simulink model "STFT_Log_IP"  (R2023b)
settings: Solver=VariableStepAuto  StartTime=0.0  StopTime=5*2*2048*15/fs  RelTol=1e-3
values from neighbouring files (symbols this model uses):
  f = 14.5e6    (= 14500000)    [startup.m]
  fs = 16e6    (= 16000000)    [startup.m]
  N = 2048    [startup.m]
libraries: hdlBasic x55, hdlDSPIP x1, hdlsllib x1, dspsrcs4 x1, vmcUtilities x1
settings Model: Creator=andre  LastModifiedBy=andre

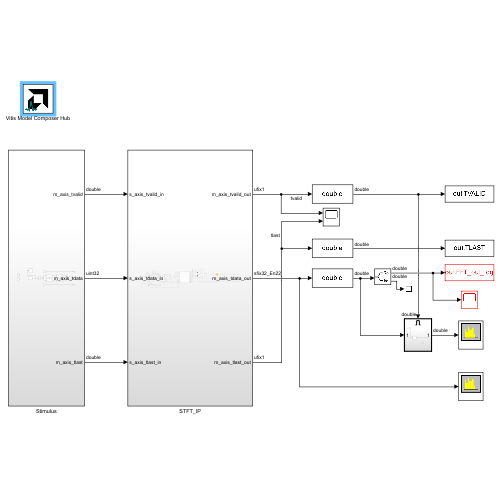
[thumbnail: Simulink's stored preview of the top-level diagram]
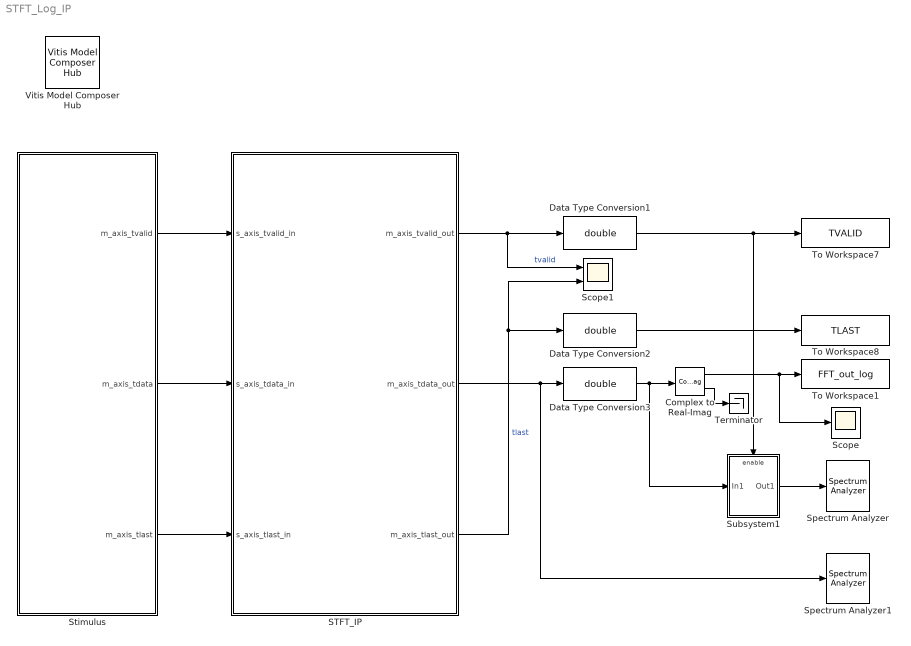
== system STFT_Log_IP ==
  Complex to Real-Imag : ComplexToRealImag
  Data Type Conversion1 : DataTypeConversion  OutDataTypeStr=double  RndMeth=Floor
  Data Type Conversion2 : DataTypeConversion  OutDataTypeStr=double  RndMeth=Floor
  Data Type Conversion3 : DataTypeConversion  OutDataTypeStr=double  RndMeth=Floor
  STFT_IP : Subsystem
  Scope : Scope
  Scope1 : Scope  NumInputPorts=2
  Spectrum Analyzer : SpectrumAnalyzer  WindowPosition=[2193.000000,-144.000000,800.000000,500.000000,]  ScopeFrameLocation=window  InputDomain=Frequency  ViewType=Spectrum and spectrogram  SampleRate=16000000  PlotAsTwoSidedSpectrum=off  AxesScaling=Manual  Span=5000  CenterFrequency=2500  StartFrequency=0  AveragingMethod=Exponential  SpectrumUnits=Auto  YLimits=[-192.92718452,-9.62777478]  ColorLimits=[-192.92718452,-9.62777478]  ExpandToolstrip=on  DefaultConfigurationName=spbscopes.SpectrumAnalyzerBlockCfg  IsFrequencyInputMode=1  FrequencyVectorPort=0  FrequencyVectorFromPort=0  FrequencyInputRBWPort=0  FrequencyInputRBWFromPort=0
  Spectrum Analyzer1 : SpectrumAnalyzer  WindowPosition=[2780.000000,-120.000000,800.000000,500.000000,]  ScopeFrameLocation=window  ViewType=Spectrum and spectrogram  SampleRate=16000000  PlotAsTwoSidedSpectrum=off  AxesScaling=Manual  Span=5000  CenterFrequency=2500  StartFrequency=0  AveragingMethod=Exponential  YLimits=[-4.45804472,88.02345412]  ColorLimits=[-4.45804472,88.02345412]  ExpandToolstrip=on  SelectedToolstripTab=spectrumAnalyzerToolstrip.estimationTab  DefaultConfigurationName=spbscopes.SpectrumAnalyzerBlockCfg  IsFrequencyInputMode=1  FrequencyVectorPort=0  FrequencyVectorFromPort=0  FrequencyInputRBWPort=0  FrequencyInputRBWFromPort=0
  Stimulus : Subsystem
  Subsystem1 : Subsystem
  Terminator : Terminator
  To Workspace1 : ToWorkspace  VariableName=FFT_out_log  SampleTime=-1
      settings: Save2DSignal=2-D array (concatenate along first dimension)
  To Workspace7 : ToWorkspace  VariableName=TVALID  SampleTime=1/fs
      settings: Save2DSignal=2-D array (concatenate along first dimension)
  To Workspace8 : ToWorkspace  VariableName=TLAST  SampleTime=1/fs
      settings: Save2DSignal=2-D array (concatenate along first dimension)
  Vitis Model Composer Hub : vmcUtilities/Vitis Model Composer Hub  Tag=genX  CodeGeneration=off  SubsystemName=STFT_IP  DUTSubsystemName=STFT_IP  CompilationType=HDLCompilation  ExportTypeV2=IP Catalog  TargetDirectory=./netlist\ip\STFT_IP\src  exportDesign=on  analyzeDesign=off  validateDesignOnHw=off  ExportType=HDL  IpVendor=xilinx.com  IpLibrary=hls  IpVersion=1.0  IpHWLanguage=Verilog  AieCompilerOptions={}  AieSimulatorOptions={}  CreateTestbench=off  TestbenchStackSize=10  RunRtlSim=off  RunCSim=off  RunAieSim=off  AieSimTimeout=50000  RunAieSimProfiling=off  LaunchVitisAnalyzer=off  PlotOutput=off  RunX86Sim=off  X86SimTimeout=10  GenHwImage=off  GenLibadfXo=on  GenHwValidationCode=off  PlatformType=Not Specified  HwSystemType=Baremetal  HwValidationTarget=hw  ProjDevice=xczu28dr-ffvg1517-2-e  ProjDevicePart=xczu28dr-ffvg1517-2-e  SamplePeriod=-1  ClockFrequency=200  DataPathParallelism=1  xilinxfamily=zynquplusRFSOC  part=xczu28dr  speed=-2-e  package=ffvg1517  directory=./netlist\ip\STFT_IP\src  testbench=off  incr_netlist=off  synthesis_tool=Vivado  clock_wrapper=Clock Enables  dbl_ovrd=According to Block Masks  dcm_input_clock_period=10  sysclk_period=(1/fs)*(1e6)  simulink_period=1/fs  eval_field=0  IPInfoJsonString="{\"HDLSubsystem\":{\"SubsystemName\":\"STFT_IP\",\"IPName\":\"STFT\",\"IPLibrary\":\"VMC\",\"IPVendor\":\"CoRSoC\",\"IPVersion\":\"1.0\",\"TargetDirectory\":\"./netlist\",\"SubsystemDir\":\"./netlist\\\\ip\\\\STFT_IP\"},\"SubsystemTag\":\"HDLNode\"}"  LogFileName=''  NThreads=4
  wires:
  Stimulus/3(m_axis_tlast) -> STFT_IP/3(s_axis_tlast_in)
  Data Type Conversion1/1 -> To Workspace7/1, Subsystem1/Enable
  Subsystem1/1(Out1) -> Spectrum Analyzer/1
  Complex to Real-Imag/2 -> Terminator/1
  Complex to Real-Imag/1 -> To Workspace1/1, Scope/1
  Data Type Conversion3/1 -> Subsystem1/1(In1), Complex to Real-Imag/1
  STFT_IP/2(m_axis_tdata_out) -> Spectrum Analyzer1/1, Data Type Conversion3/1
  STFT_IP/3(m_axis_tlast_out) -> Scope1/2, Data Type Conversion2/1  "tlast"
  STFT_IP/1(m_axis_tvalid_out) -> Data Type Conversion1/1, Scope1/1  "tvalid"
  Data Type Conversion2/1 -> To Workspace8/1
  Stimulus/1(m_axis_tvalid) -> STFT_IP/1(s_axis_tvalid_in)
  Stimulus/2(m_axis_tdata) -> STFT_IP/2(s_axis_tdata_in)

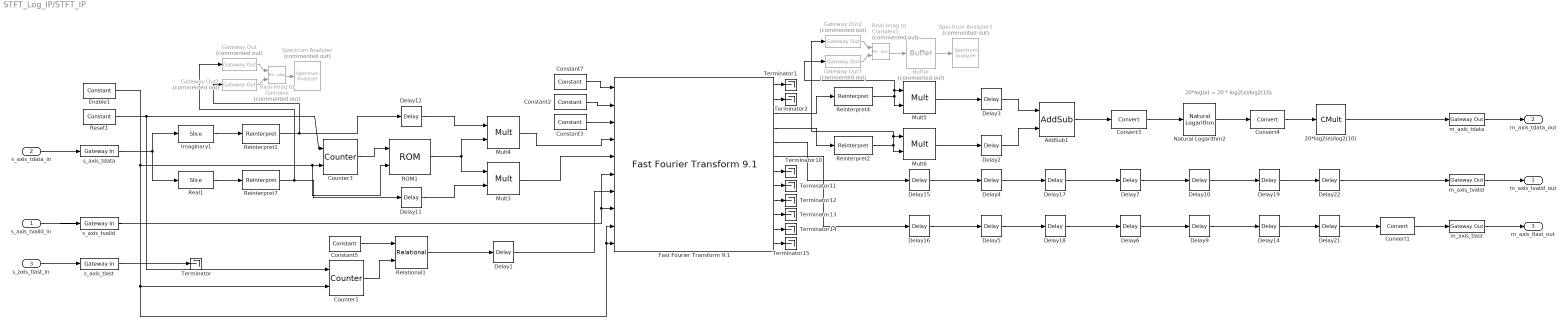
== system STFT_Log_IP/STFT_IP ==
  note: 20*log(x) = 20 * log2(x)/log2(10)
  s_axis_tvalid_in : Inport
  s_axis_tdata_in : Inport  Port=2
  s_axis_tlast_in : Inport  Port=3
  20*log2(e)/log2(10) : hdlBasic/CMult  const=20*1.44269504089/3.32192809489  gui_display_data_type=Fixed-point  const_n_bits=20  const_bin_pt=16  float_type=Single  exp_bits=8  fraction_bits=24  en=off  latency=2  precision=User Defined  arith_type="Signed  (2's comp)"  n_bits=32  bin_pt=32-10  quantization=Truncate  overflow=Saturate  use_behavioral_HDL=off  mem_type=Distributed RAM  pipeline=off  XmcBlockStatus=1  maskContainerNames=tabcontainer1  block_type=cmult  block_config=sysgen:CMult_config
      settings: infoedit=[]
  AddSub1 : hdlBasic/AddSub  mode=Addition  use_carryin=off  use_carryout=off  en=off  latency=1  precision=User Defined  arith_type="Signed  (2's comp)"  n_bits=32  bin_pt=29  quantization=Truncate  overflow=Saturate  use_behavioral_HDL=off  hw_selection=Fabric  pipelined=off  XmcBlockStatus=1  maskContainerNames=tabcontainer1  block_type=addsub  block_config=sysgen:Addsub_config
  Buffer : Buffer  Commented=on  OutputFrames=off
  Constant2 : hdlBasic/Constant  const=0  gui_display_data_type=Fixed-point  arith_type=Unsigned  n_bits=1  bin_pt=0  preci_type=Single  exp_width=8  frac_width=24  explicit_period=on  period=1/fs  XmcBlockStatus=1  maskContainerNames=tabcontainer1  block_type=constant  block_config=sysgen:Constant_config
  Constant3 : hdlBasic/Constant  const=0  gui_display_data_type=Boolean  arith_type=Boolean  n_bits=1  bin_pt=0  preci_type=Single  exp_width=8  frac_width=24  explicit_period=on  period=1/fs  XmcBlockStatus=1  maskContainerNames=tabcontainer1  block_type=constant  block_config=sysgen:Constant_config
  Constant5 : hdlBasic/Constant  const=N-1  gui_display_data_type=Fixed-point  arith_type=Unsigned  n_bits=11  bin_pt=0  preci_type=Single  exp_width=8  frac_width=24  explicit_period=on  period=1/fs  XmcBlockStatus=1  maskContainerNames=tabcontainer1  block_type=constant  block_config=sysgen:Constant_config
  Constant7 : hdlBasic/Constant  const=0  gui_display_data_type=Fixed-point  arith_type=Unsigned  n_bits=12  bin_pt=0  preci_type=Single  exp_width=8  frac_width=24  explicit_period=on  period=1/fs  XmcBlockStatus=1  maskContainerNames=tabcontainer1  block_type=constant  block_config=sysgen:Constant_config
  Convert1 : hdlBasic/Convert  gui_display_data_type=Boolean  arith_type=Boolean  n_bits=16  bin_pt=14  float_type=Single  exp_bits=8  fraction_bits=24  quantization=Truncate  overflow=Wrap  en=off  latency=0  pipeline=off  XmcBlockStatus=1  maskContainerNames=group2  block_type=convert  block_config=sysgen:Convert_config  block_width=595  block_height=885
  Convert3 : hdlBasic/Convert  gui_display_data_type=Floating-point  arith_type=Floating-point  n_bits=16  bin_pt=14  float_type=Single  exp_bits=8  fraction_bits=24  quantization=Truncate  overflow=Wrap  en=off  latency=1  pipeline=off  XmcBlockStatus=1  maskContainerNames=group2  block_type=convert  block_config=sysgen:Convert_config  block_width=595  block_height=885
  Convert4 : hdlBasic/Convert  gui_display_data_type=Fixed-point  arith_type="Signed  (2's comp)"  n_bits=32  bin_pt=32-10  float_type=Single  exp_bits=8  fraction_bits=24  quantization="Round  (unbiased: +/- Inf)"  overflow=Saturate  en=off  latency=1  pipeline=off  XmcBlockStatus=1  maskContainerNames=group2  block_type=convert  block_config=sysgen:Convert_config  block_width=595  block_height=885
  Counter1 : hdlBasic/Counter  cnt_type=Count limited  cnt_to=N-1  operation=Up  start_count=0  cnt_by_val=1  arith_type=Unsigned  n_bits=11  bin_pt=0  load_pin=off  rst=on  en=on  explicit_period=Explicit  period=1/fs  use_behavioral_HDL=off  implementation=Fabric  XmcBlockStatus=1  maskContainerNames=group1  block_type=counter  block_config=sysgen:Counter_config  block_width=531  block_height=1023
  Counter3 : hdlBasic/Counter  cnt_type=Count limited  cnt_to=N-1  operation=Up  start_count=0  cnt_by_val=1  arith_type=Unsigned  n_bits=ceil(log2(N))  bin_pt=0  load_pin=off  rst=on  en=on  explicit_period=Explicit  period=1/fs  use_behavioral_HDL=off  implementation=Fabric  XmcBlockStatus=1  maskContainerNames=group1  block_type=counter  block_config=sysgen:Counter_config  block_width=531  block_height=1023
  Delay1 : hdlBasic/Delay  rst=off  en=off  latency=3  reg_retiming=off  XmcBlockStatus=1  maskContainerNames=group1  block_type=delay  block_config=sysgen:Delay_config
  Delay{2..7,9..12,14,17..19} (14 alike) : hdlBasic/Delay  rst=off  en=off  latency=1  reg_retiming=off  XmcBlockStatus=1  maskContainerNames=group1  block_type=delay  block_config=sysgen:Delay_config
  Delay15 : hdlBasic/Delay  rst=off  en=off  latency=3  reg_retiming=off  XmcBlockStatus=1  maskContainerNames=group1  block_type=delay  block_config=sysgen:Delay_config
  Delay16 : hdlBasic/Delay  rst=off  en=off  latency=3  reg_retiming=off  XmcBlockStatus=1  maskContainerNames=group1  block_type=delay  block_config=sysgen:Delay_config
  Delay21 : hdlBasic/Delay  rst=off  en=off  latency=2  reg_retiming=off  XmcBlockStatus=1  maskContainerNames=group1  block_type=delay  block_config=sysgen:Delay_config
  Delay22 : hdlBasic/Delay  rst=off  en=off  latency=2  reg_retiming=off  XmcBlockStatus=1  maskContainerNames=group1  block_type=delay  block_config=sysgen:Delay_config
  Enable1 : hdlBasic/Constant  const=1  gui_display_data_type=Boolean  arith_type=Boolean  n_bits=11  bin_pt=0  preci_type=Single  exp_width=8  frac_width=24  explicit_period=on  period=1/fs  XmcBlockStatus=1  maskContainerNames=tabcontainer1  block_type=constant  block_config=sysgen:Constant_config
  Fast Fourier Transform 9.1 : hdlDSPIP/Fast Fourier Transform 9.1   transform_length=2048  target_clock_frequency=64  target_data_throughput=50  implementation_options=pipelined_streaming_io  run_time_configurable_transform_length=off  phase_factor_width=16  scaling_options=scaled  rounding_modes=truncation  aclken=on  aresetn=on  output_ordering=natural_order  cyclic_prefix_insertion=off  throttle_scheme=nonrealtime  xk_index=off  ovflo=off  trim_axipin_name=on  memory_options_data=block_ram  memory_options_phase_factors=block_ram  number_of_stages_using_block_ram_for_data_and_phase_factors=6  memory_options_reorder=block_ram  memory_options_hybrid=off  complex_mult_type=use_mults_resources  butterfly_type=use_luts  simulation_type=hybrid_sim  simulation_model=sysgen:xfftv9_cmodel  data_path_portlist={ 's_axis_data_tdata', 'm_axis_data_tdata', 'm_axis_status_tdata', 'event_fft_overflow' }  channels=1  input_ordering=natural_order  input_width=16  ip_name=Fast Fourier Transform  ip_version=9.1  dsptool_ready=true  ipcore_usecache=true  ipcore_useipmodelcache=true  wrapper_available=true  port_translation_map={ 'aclken' => 'en', 'aresetn' => 'rst'}  data_format=fixed_point  XmcBlockStatus=1  maskContainerNames=tabcontainer1  block_type=xfft_v9_1  block_config=sysgen:rodinimport_config
  Gateway Out{,1..3} (4 alike) : hdlBasic/Gateway Out  Commented=on  inherit_from_input=off  hdl_port=off  rows=1  columns=1  UseAsDAC=off  DACChannel='1'  interface=None  automatic_assignment=on  address_offset=hex2dec('00')  intf_name=''  intf_description=''  timing_constraint=None  locs_specified=off  LOCs={}  io_standard={}  XmcBlockStatus=1  maskContainerNames=group4  block_type=gatewayout  block_config=sysgen:gateway_out_config  block_width_w=590  block_height_w=620  block_width=620  block_height=750
  Imaginary1 : hdlBasic/Slice  nbits=16  boolean_output=off  mode=Two Bit Locations  bit1=31  base1=LSB of Input  bit0=16  base0=LSB of Input  XmcBlockStatus=1  maskContainerNames=group1  block_type=slice  block_config=sysgen:Slice_config
  Mult3 : hdlBasic/Mult  precision=User Defined  arith_type="Signed  (2's comp)"  n_bits=16  bin_pt=15  quantization=Truncate  overflow=Saturate  en=off  latency=3  use_behavioral_HDL=off  opt=Speed  use_embedded=on  optimum_pipeline=off  pipeline=on  use_rpm=on  placement_style=Triangular  XmcBlockStatus=1  maskContainerNames=group1  block_type=mult  block_config=sysgen:Mult_config  block_width=598  block_height=876
  Mult4 : hdlBasic/Mult  precision=User Defined  arith_type="Signed  (2's comp)"  n_bits=16  bin_pt=15  quantization=Truncate  overflow=Saturate  en=off  latency=3  use_behavioral_HDL=off  opt=Speed  use_embedded=on  optimum_pipeline=off  pipeline=on  use_rpm=on  placement_style=Triangular  XmcBlockStatus=1  maskContainerNames=group1  block_type=mult  block_config=sysgen:Mult_config  block_width=598  block_height=876
  Mult5 : hdlBasic/Mult  precision=User Defined  arith_type=Unsigned  n_bits=32  bin_pt=31  quantization=Truncate  overflow=Saturate  en=off  latency=3  use_behavioral_HDL=off  opt=Speed  use_embedded=on  optimum_pipeline=off  pipeline=on  use_rpm=on  placement_style=Triangular  XmcBlockStatus=1  maskContainerNames=group1  block_type=mult  block_config=sysgen:Mult_config  block_width=598  block_height=876
  Mult6 : hdlBasic/Mult  precision=User Defined  arith_type=Unsigned  n_bits=32  bin_pt=31  quantization=Truncate  overflow=Saturate  en=off  latency=3  use_behavioral_HDL=off  opt=Speed  use_embedded=on  optimum_pipeline=off  pipeline=on  use_rpm=on  placement_style=Triangular  XmcBlockStatus=1  maskContainerNames=group1  block_type=mult  block_config=sysgen:Mult_config  block_width=598  block_height=876
  Natural Logarithm2 : hdlBasic/Natural Logarithm  flow_control=NonBlocking  axi_optimize_goal=Resources  latency=1  has_a_tlast=off  has_a_tuser=off  en=off  has_result_tready=off  has_invalid_op=off  has_divide_by_zero=off  fpo_op_type=log_base_e  rate=1  has_b_tlast=false  has_b_tuser=false  result_tlast_behv=1  has_underflow=false  has_overflow=false  XmcBlockStatus=1  maskContainerNames=tabcontainer1  block_type=natlog  block_config=sysgen:FPOBlockDescriptor_config
  ROM1 : hdlBasic/ROM  depth=N  initVector=Hanning  distributed_mem=Block RAM  rst=off  init_reg=0  en=on  latency=1  gui_display_data_type=Fixed-point  arith_type=Unsigned  n_bits=16  bin_pt=15  preci_type=Single  exp_width=8  frac_width=24  optimize=Area  use_rpm=on  simulation_type=fast_sim  XmcBlockStatus=1  maskContainerNames=tabcontainer1  block_type=sprom  block_config=sysgen:SPROM_config
  Real-Imag to Complex : RealImagToComplex  Commented=on
  Real-Imag to Complex1 : RealImagToComplex  Commented=on
  Real1 : hdlBasic/Slice  nbits=16  boolean_output=off  mode=Two Bit Locations  bit1=15  base1=LSB of Input  bit0=0  base0=LSB of Input  XmcBlockStatus=1  maskContainerNames=group1  block_type=slice  block_config=sysgen:Slice_config
  Reinterpret1 : hdlBasic/Reinterpret  force_arith_type=on  arith_type="Signed  (2's comp)"  force_bin_pt=on  bin_pt=15  XmcBlockStatus=1  maskContainerNames=group1  block_type=reinterpret  block_config=sysgen:Reinterpret_config
  Reinterpret2 : hdlBasic/Reinterpret  force_arith_type=on  arith_type="Signed  (2's comp)"  force_bin_pt=off  bin_pt=31  XmcBlockStatus=1  maskContainerNames=group1  block_type=reinterpret  block_config=sysgen:Reinterpret_config
  Reinterpret4 : hdlBasic/Reinterpret  force_arith_type=on  arith_type="Signed  (2's comp)"  force_bin_pt=off  bin_pt=31  XmcBlockStatus=1  maskContainerNames=group1  block_type=reinterpret  block_config=sysgen:Reinterpret_config
  Reinterpret7 : hdlBasic/Reinterpret  force_arith_type=on  arith_type="Signed  (2's comp)"  force_bin_pt=on  bin_pt=15  XmcBlockStatus=1  maskContainerNames=group1  block_type=reinterpret  block_config=sysgen:Reinterpret_config
  Relational1 : hdlBasic/Relational  mode=a=b  op_type=Bool  en=off  latency=1  XmcBlockStatus=1  maskContainerNames=tabcontainer1  block_type=relational  block_config=sysgen:Relational_config
  Reset1 : hdlBasic/Constant  const=0  gui_display_data_type=Boolean  arith_type=Boolean  n_bits=11  bin_pt=0  preci_type=Single  exp_width=8  frac_width=24  explicit_period=on  period=1/fs  XmcBlockStatus=1  maskContainerNames=tabcontainer1  block_type=constant  block_config=sysgen:Constant_config
  Spectrum Analyzer : SpectrumAnalyzer  Commented=on  WindowPosition=[323.000000,106.000000,800.000000,500.000000,]  ScopeFrameLocation=window  Span=16000000  StartFrequency=-8000000  StopFrequency=8000000  YLimits=[-214.59627124,48.33447167]
  Spectrum Analyzer1 : SpectrumAnalyzer  Commented=on  WindowPosition=[323.000000,106.000000,800.000000,500.000000,]  ScopeFrameLocation=window  InputDomain=Frequency  Span=16000000  StartFrequency=-8000000  StopFrequency=8000000  SpectrumUnits=Auto  YLimits=[-0.00003052,0]  SelectedToolstripTab=spectrumAnalyzerToolstrip.measurementsTab
  Terminator{,1..2,10..15} (9 alike) : Terminator
  m_axis_tdata : hdlBasic/Gateway Out  inherit_from_input=on  hdl_port=on  rows=1  columns=1  UseAsDAC=off  DACChannel='1'  interface=None  automatic_assignment=on  address_offset=hex2dec('00')  intf_name=''  intf_description=''  timing_constraint=None  locs_specified=off  LOCs={}  io_standard={}  XmcBlockStatus=1  maskContainerNames=group4  block_type=gatewayout  block_config=sysgen:gateway_out_config  block_width_w=590  block_height_w=620  block_width=620  block_height=750
  m_axis_tlast : hdlBasic/Gateway Out  inherit_from_input=on  hdl_port=on  rows=1  columns=1  UseAsDAC=off  DACChannel='1'  interface=None  automatic_assignment=on  address_offset=hex2dec('00')  intf_name=''  intf_description=''  timing_constraint=None  locs_specified=off  LOCs={}  io_standard={}  XmcBlockStatus=1  maskContainerNames=group4  block_type=gatewayout  block_config=sysgen:gateway_out_config  block_width_w=590  block_height_w=620  block_width=620  block_height=750
  m_axis_tvalid : hdlBasic/Gateway Out  inherit_from_input=on  hdl_port=on  rows=1  columns=1  UseAsDAC=off  DACChannel='1'  interface=None  automatic_assignment=on  address_offset=hex2dec('00')  intf_name=''  intf_description=''  timing_constraint=None  locs_specified=off  LOCs={}  io_standard={}  XmcBlockStatus=1  maskContainerNames=group4  block_type=gatewayout  block_config=sysgen:gateway_out_config  block_width_w=590  block_height_w=620  block_width=620  block_height=750
  s_axis_tdata : hdlBasic/Gateway In  gui_display_data_type=Fixed-point  arith_type=Unsigned  n_bits=32  bin_pt=0  preci_type=Single  exp_width=8  frac_width=24  rows=1  columns=1  quantization="Round  (unbiased: +/- Inf)"  overflow=Saturate  period=1/fs  UseAsADC=off  ADCChannel='1'  interface=None  automatic_assignment=on  address_offset=hex2dec('00')  intf_name=''  intf_description=''  default_value=0  timing_constraint=None  locs_specified=off  LOCs={}  io_standard={}  inherit_from_input=off  hdl_port=on  XmcBlockStatus=1  maskContainerNames=group4  block_type=gatewayin  block_config=sysgen:gateway_in_config  block_width_w=590  block_height_w=620  block_width=640  block_height=850
  s_axis_tlast : hdlBasic/Gateway In  gui_display_data_type=Boolean  arith_type=Boolean  n_bits=16  bin_pt=14  preci_type=Single  exp_width=8  frac_width=24  rows=1  columns=1  quantization="Round  (unbiased: +/- Inf)"  overflow=Saturate  period=1/fs  UseAsADC=off  ADCChannel='1'  interface=None  automatic_assignment=on  address_offset=hex2dec('00')  intf_name=''  intf_description=''  default_value=0  timing_constraint=None  locs_specified=off  LOCs={}  io_standard={}  inherit_from_input=off  hdl_port=on  XmcBlockStatus=1  maskContainerNames=group4  block_type=gatewayin  block_config=sysgen:gateway_in_config  block_width_w=590  block_height_w=620  block_width=640  block_height=850
  s_axis_tvalid : hdlBasic/Gateway In  gui_display_data_type=Boolean  arith_type=Boolean  n_bits=16  bin_pt=14  preci_type=Single  exp_width=8  frac_width=24  rows=1  columns=1  quantization="Round  (unbiased: +/- Inf)"  overflow=Saturate  period=1/fs  UseAsADC=off  ADCChannel='1'  interface=None  automatic_assignment=on  address_offset=hex2dec('00')  intf_name=''  intf_description=''  default_value=0  timing_constraint=None  locs_specified=off  LOCs={}  io_standard={}  inherit_from_input=off  hdl_port=on  XmcBlockStatus=1  maskContainerNames=group4  block_type=gatewayin  block_config=sysgen:gateway_in_config  block_width_w=590  block_height_w=620  block_width=640  block_height=850
  m_axis_tvalid_out : Outport
  m_axis_tdata_out : Outport  Port=2
  m_axis_tlast_out : Outport  Port=3
  wires:
  s_axis_tlast_in/1 -> s_axis_tlast/1
  Imaginary1/1 -> Reinterpret1/1
  Delay12/1 -> Mult4/1
  Fast Fourier Transform 9.1/11 -> Terminator14/1
  Delay16/1 -> Delay5/1
  Constant3/1 -> Fast Fourier Transform 9.1/3
  Relational1/1 -> Delay1/1
  Delay1/1 -> Fast Fourier Transform 9.1/7
  Delay11/1 -> Mult3/2
  Counter1/1 -> Relational1/2
  Constant5/1 -> Relational1/1
  Fast Fourier Transform 9.1/2 -> Terminator2/1
  Fast Fourier Transform 9.1/1 -> Terminator1/1
  s_axis_tdata_in/1 -> s_axis_tdata/1
  Fast Fourier Transform 9.1/3 -> Reinterpret4/1
  Fast Fourier Transform 9.1/10 -> Terminator13/1
  Mult6/1 -> Delay2/1
  Fast Fourier Transform 9.1/7 -> Terminator10/1
  Mult4/1 -> Fast Fourier Transform 9.1/4
  Reinterpret4/1 -> Gateway Out3/1, Mult5/1, Mult5/2
  Reinterpret2/1 -> Gateway Out2/1, Mult6/1, Mult6/2
  Delay15/1 -> Delay4/1
  ROM1/1 -> Mult4/2, Mult3/1
  Fast Fourier Transform 9.1/8 -> Terminator11/1
  Fast Fourier Transform 9.1/12 -> Terminator15/1
  Counter3/1 -> ROM1/1
  Fast Fourier Transform 9.1/6 -> Delay16/1
  Constant2/1 -> Fast Fourier Transform 9.1/2
  Real1/1 -> Reinterpret7/1
  Fast Fourier Transform 9.1/9 -> Terminator12/1
  Fast Fourier Transform 9.1/4 -> Reinterpret2/1
  Mult5/1 -> Delay3/1
  s_axis_tvalid_in/1 -> s_axis_tvalid/1
  Reinterpret1/1 -> Gateway Out1/1, Delay12/1
  Enable1/1 -> Counter3/2, ROM1/2, Counter1/2, Fast Fourier Transform 9.1/10, Fast Fourier Transform 9.1/9
  Reinterpret7/1 -> Gateway Out/1, Delay11/1
  Reset1/1 -> Counter1/1, Counter3/1
  Delay18/1 -> Delay6/1
  Mult3/1 -> Fast Fourier Transform 9.1/5
  Convert1/1 -> m_axis_tlast/1
  Delay2/1 -> AddSub1/2
  Delay3/1 -> AddSub1/1
  Delay4/1 -> Delay17/1
  Delay5/1 -> Delay18/1
  Constant7/1 -> Fast Fourier Transform 9.1/1
  s_axis_tvalid/1 -> Fast Fourier Transform 9.1/6, Fast Fourier Transform 9.1/8
  s_axis_tdata/1 -> Real1/1, Imaginary1/1
  s_axis_tlast/1 -> Terminator/1
  m_axis_tdata/1 -> m_axis_tdata_out/1
  m_axis_tvalid/1 -> m_axis_tvalid_out/1
  m_axis_tlast/1 -> m_axis_tlast_out/1
  Delay17/1 -> Delay7/1
  Fast Fourier Transform 9.1/5 -> Delay15/1
  AddSub1/1 -> Convert3/1
  Convert3/1 -> Natural Logarithm2/1
  Natural Logarithm2/1 -> Convert4/1
  Convert4/1 -> 20*log2(e)/log2(10)/1
  Delay6/1 -> Delay9/1
  Delay7/1 -> Delay10/1
  Delay9/1 -> Delay14/1
  Delay10/1 -> Delay19/1
  Delay14/1 -> Delay21/1
  Delay19/1 -> Delay22/1
  Delay21/1 -> Convert1/1
  Delay22/1 -> m_axis_tvalid/1
  20*log2(e)/log2(10)/1 -> m_axis_tdata/1
  Real-Imag to Complex/1 -> Spectrum Analyzer/1
  Gateway Out/1 -> Real-Imag to Complex/1
  Gateway Out1/1 -> Real-Imag to Complex/2
  Gateway Out3/1 -> Real-Imag to Complex1/2
  Gateway Out2/1 -> Real-Imag to Complex1/1
  Real-Imag to Complex1/1 -> Buffer/1
  Buffer/1 -> Spectrum Analyzer1/1

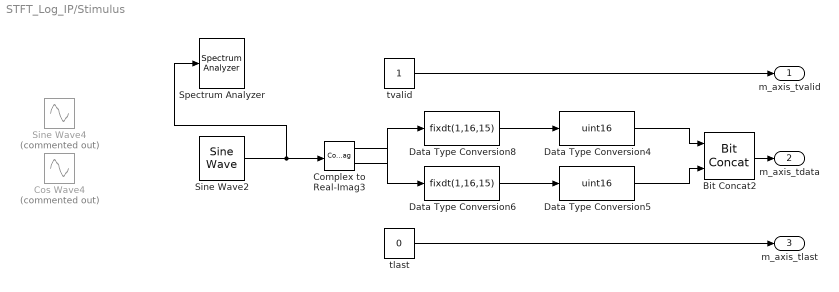
== system STFT_Log_IP/Stimulus ==
  Bit Concat2 : hdlsllib/Logic and Bit Operations/Bit Concat  numInputs=2
  Complex to Real-Imag3 : ComplexToRealImag
  Cos Wave4 : Sin  Commented=on  Amplitude=0.4  Frequency=f*pi  Phase=pi/2  SampleTime=1/fs
  Data Type Conversion4 : DataTypeConversion  OutDataTypeStr=uint16  ConvertRealWorld=Stored Integer (SI)  SaturateOnIntegerOverflow=off  RndMeth=Floor
  Data Type Conversion5 : DataTypeConversion  OutDataTypeStr=uint16  ConvertRealWorld=Stored Integer (SI)  SaturateOnIntegerOverflow=off  RndMeth=Floor
  Data Type Conversion6 : DataTypeConversion  OutDataTypeStr=fixdt(1,16,15)  RndMeth=Floor
  Data Type Conversion8 : DataTypeConversion  OutDataTypeStr=fixdt(1,16,15)  RndMeth=Floor
  Sine Wave2 : dspsrcs4/Sine Wave  Amplitude=0.4  Frequency=f  Phase=0  SampleMode=Discrete  OutComplex=Complex  CompMethod=Trigonometric fcn  TableSize=Speed  SampleTime=1/(fs)  SamplesPerFrame=1  ResetState=Restart at time zero  OutputFrames=off  dataType=double  wordLen=16  udDataType=sfix(16)  fracBitsMode=Best precision  numFracBits=15  OutDataTypeStr=double  LastOutDataTypeStr=double
  Sine Wave4 : Sin  Commented=on  Amplitude=0.4  Frequency=f*pi  SampleTime=1/fs
  Spectrum Analyzer : SpectrumAnalyzer  WindowPosition=[2272.000000,-134.000000,800.000000,500.000000,]  ScopeFrameLocation=window  Span=128000000  StartFrequency=-64000000  StopFrequency=64000000  YLimits=[-214.54105276,48.32811539]
  tlast : Constant  Value=0  SampleTime=1/fs
  tvalid : Constant  SampleTime=1/fs
  m_axis_tvalid : Outport
  m_axis_tdata : Outport  Port=2
  m_axis_tlast : Outport  Port=3
  wires:
  Data Type Conversion6/1 -> Data Type Conversion5/1
  Data Type Conversion4/1 -> Bit Concat2/1
  Data Type Conversion8/1 -> Data Type Conversion4/1
  Data Type Conversion5/1 -> Bit Concat2/2
  Bit Concat2/1 -> m_axis_tdata/1
  tvalid/1 -> m_axis_tvalid/1
  tlast/1 -> m_axis_tlast/1
  Sine Wave2/1 -> Spectrum Analyzer/1, Complex to Real-Imag3/1
  Complex to Real-Imag3/1 -> Data Type Conversion6/1
  Complex to Real-Imag3/2 -> Data Type Conversion8/1

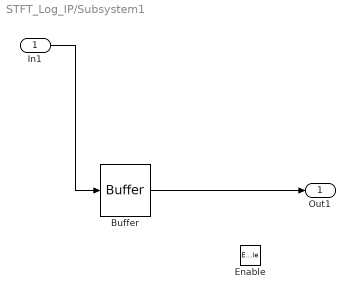
== system STFT_Log_IP/Subsystem1 ==
  In1 : Inport
  Enable : EnablePort
  Buffer : Buffer  N=2048  OutputFrames=off
  Out1 : Outport
  wires:
  In1/1 -> Buffer/1
  Buffer/1 -> Out1/1
